simulink model "arm"  (R2016b)
settings: Solver=VariableStepAuto  StartTime=0.0  StopTime=120  RelTol=1e-3
settings Model: Creator=Dorry Cao  LastModifiedBy=Dorry Cao

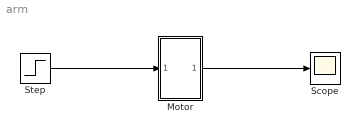
== system arm ==
  Motor : Subsystem
  Scope : Scope
  Step : Step  SampleTime=0
  wires:
  Motor/1(Out1) -> Scope/1
  Step/1 -> Motor/1(In1)

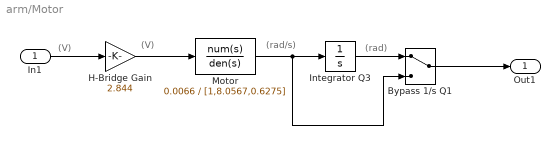
== system arm/Motor ==
  note: (rad)
  note: (V)
  note: (rad/s)
  note: (V)
  In1 : Inport
  Bypass 1/s Q1 : ManualSwitch
  H-Bridge Gain : Gain  Gain=2.844
  Integrator Q3 : Integrator
  "Motor " : TransferFcn  Numerator=0.0066  Denominator=[1,8.0567,0.6275]
  Out1 : Outport
  wires:
  "Motor "/1 -> Bypass 1/s Q1/2, Integrator Q3/1
  H-Bridge Gain/1 -> "Motor "/1
  In1/1 -> H-Bridge Gain/1
  Integrator Q3/1 -> Bypass 1/s Q1/1
  Bypass 1/s Q1/1 -> Out1/1
